simulink model "Temp"  (R2024b)
settings: Solver=VariableStepAuto  StartTime=0.0  StopTime=10.0  RelTol=1e-3
libraries: simulink x4
settings Model: Creator=idrin  LastModifiedBy=idrin

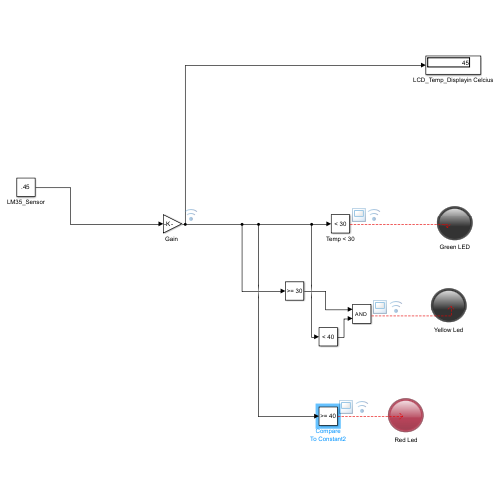
[thumbnail: Simulink's stored preview of the top-level diagram]
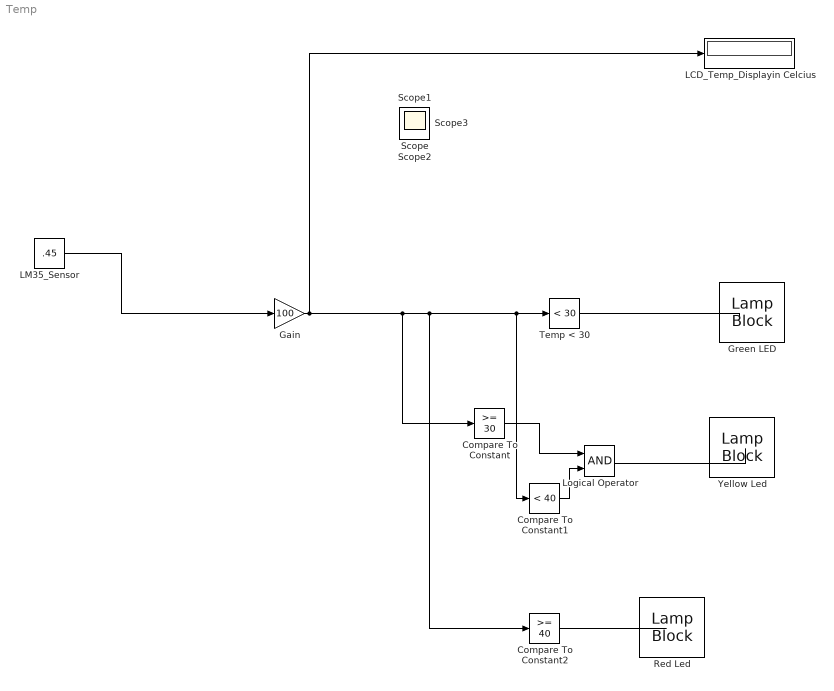
== system Temp ==
  Compare To Constant : simulink/Logic and Bit Operations/Compare To Constant  relop=>=  const=30  OutDataTypeStr=boolean
  Compare To Constant1 : simulink/Logic and Bit Operations/Compare To Constant  relop=<  const=40  OutDataTypeStr=boolean
  Compare To Constant2 : simulink/Logic and Bit Operations/Compare To Constant  relop=>=  const=40  OutDataTypeStr=boolean
  "Gain " : Gain  Gain=100
  Green LED : LampBlock  LabelPosition=Hide
  LCD_Temp_Displayin Celcius : Display
  LM35_Sensor : Constant  Value=.45
  Logical Operator : Logic  OutDataTypeStr=boolean
  Red Led : LampBlock  LabelPosition=Hide
  Temp < 30 : simulink/Logic and Bit Operations/Compare To Constant  relop=<  const=30  OutDataTypeStr=boolean
  Yellow Led : LampBlock  LabelPosition=Hide
  Scope{,1..3} (4 alike) : Scope
  wires:
  LM35_Sensor/1 -> "Gain "/1
  Compare To Constant/1 -> Logical Operator/1
  Compare To Constant1/1 -> Logical Operator/2
  "Gain "/1 -> LCD_Temp_Displayin Celcius/1, Compare To Constant1/1, Temp < 30/1, Compare To Constant2/1, Compare To Constant/1
  Temp < 30/1 -> ?
  Logical Operator/1 -> ?
  Compare To Constant2/1 -> ?
